simulink model "SF049A_LoaMgr"  (R2013b)
settings: Solver=FixedStepDiscrete  SolverMode=SingleTasking  StartTime=0.0  StopTime=1  FixedStep=0.002  RelTol=1e-3
undefined symbols (not defined in the file): CURRMEASLOAMTGTNMASK_CNT_U08, IVTRLOAMTGTNMASK_CNT_U08, LoaCtrldShtdwn, LoaCurrMeasIdptSigNrFlt, LoaHwTqIdptSigNrFlt, LoaImdtShtdwn, LoaIvtrIdptSigNrFlt, LOAMAXSLEW_ULSPERSEC_F32, LoaMgrCurrIvtrMtgtnRate, LoaMgrCurrIvtrMtgtnSca, LoaMgrCurrIvtrMtgtnScaZeroEna, LoaMgrCurrMeasIdptSig0Resp, LoaMgrCurrMeasIdptSig1Resp, LoaMgrCurrMeasIdptSig2Resp, LoaMgrCurrMeasIdptSigFltThd, LoaMgrCurrMeasMtgtnRate, LoaMgrCurrMeasMtgtnSca, LoaMgrCurrMeasMtgtnScaZeroEna, LoaMgrFadeOutStRate, LoaMgrHwTqIdptSig0NoTqLoaResp, LoaMgrHwTqIdptSig1NoTqLoaResp, LoaMgrHwTqIdptSig2Resp, LoaMgrHwTqIdptSig4Resp, LoaMgrHwTqIdptSigFltThd, LoaMgrHwTqLoaAvlResp, LoaMgrIvtrIdptSig0Resp, LoaMgrIvtrIdptSig1Resp, LoaMgrIvtrIdptSig2Resp, LoaMgrIvtrIdptSigFltThd, LoaMgrIvtrMtgtnRate, LoaMgrIvtrMtgtnSca, LoaMgrIvtrMtgtnScaZeroEna, LoaMgrLimdStRate, LoaMgrLimdStSca, LoaMgrMotAgAvlSnsrlsResp, LoaMgrMotAgIdptSig0NoSnsrlsResp, LoaMgrMotAgIdptSig1NoSnsrlsResp, LoaMgrMotAgIdptSig2Resp, LoaMgrMotAgIdptSig3Resp, LoaMgrMotAgIdptSigFltThd, LoaMgrMotAgMtgtnRate, LoaMgrMotAgMtgtnSca, LoaMgrMotAgMtgtnScaZeroEna, LoaMotAgIdptSigNrFlt, LOASCAONE_ULS_F32, LOASCAZERO_ULS_F32, LoaSt1, LOASTIMDTSHTDWN_CNT_U08, LOASTNORM_CNT_U08, LOASTSWMTGTN_CNT_U08, MAXCURRMEASIDPTSIGALLWD_CNT_U08, MAXHWTQIDPTSIGALLWD_CNT_U08, MAXIVTRIDPTSIGALLWD_CNT_U08, MAXMOTAGMECLIDPTSIGALLWD_CNT_U08, NODEBSTEP_CNT_U16, NtcSts1, SigQlfr1
libraries: simulink x30, NxtrMin x4, NxtrMax x4, NxtrLim x2
(part 4 of 7)

== system SF049A_LoaMgr/LoaMgr/LoaMgrPer1/Arbitrate_Responses/SelFinalResp ==
  note: Pick the most severe of all the requested responses.
      |
      | 5 Immediate Shutdown  (most severe)
      | 4 Controlled Shutdown
      | 3 FadeOut
      | 2 Software-based Mitigation
      | 1 Reduced Performance
      | 0 Normal Operation       (least severe)
  note: Set case 5 as the default.
  MultiMtgtnResp : Inport  RequirementInfo="{'linktype_rmi_doors' '00012fd5 (/E-STEER Core/SubSystem Specifications/Application Functions - EA4/SF049A Loss of Assist Manager)' '#SF049A_145' 'true' 'REQ:  SF049A_145' '' } %GIDa_0bea4813_eb32_4058_8f76_4a113310606c"
  HwTqResp : Inport  RequirementInfo="{'linktype_rmi_doors' '00012fd5 (/E-STEER Core/SubSystem Specifications/Application Functions - EA4/SF049A Loss of Assist Manager)' '#SF049A_145' 'true' 'REQ:  SF049A_145' '' } %GIDa_fb7392d9_74f6_4982_b9b2_ff40e0228010"  Port=2
  MotAgResp : Inport  RequirementInfo="{'linktype_rmi_doors' '00012fd5 (/E-STEER Core/SubSystem Specifications/Application Functions - EA4/SF049A Loss of Assist Manager)' '#SF049A_145' 'true' 'REQ:  SF049A_145' '' } %GIDa_e26ca98c_5988_46fe_9836_793f54528b6a"  Port=3
  CurrMeasResp : Inport  RequirementInfo="{'linktype_rmi_doors' '00012fd5 (/E-STEER Core/SubSystem Specifications/Application Functions - EA4/SF049A Loss of Assist Manager)' '#SF049A_145' 'true' 'REQ:  SF049A_145' '' } %GIDa_907ff0d5_2f07_4379_9f02_e91fd766cda4"  Port=4
  IvtrResp : Inport  RequirementInfo="{'linktype_rmi_doors' '00012fd5 (/E-STEER Core/SubSystem Specifications/Application Functions - EA4/SF049A Loss of Assist Manager)' '#SF049A_145' 'true' 'REQ:  SF049A_145' '' } %GIDa_a6dc34e3_dd60_490f_b49f_75bf24068ace"  Port=5
  CopyRight2 : Subsystem  Description=|  mask(Copyright Information){none=on}
      | Copyright info block.                                               
      |                                                                     
      | Place copyright information at the top of every subsystem in design.
      mask prompts: none "No parameters"
      mask help: Place copyright information at the top of every subsystem in design.
      mask Display:
      | NxtrConf = 'Nexteer Confidential';
      | 
      | sys = bdroot; %handle for the current model ("system")
      | first = get_param(sys,'Created');
      | first = first(end-3:end);  %year is last four digits
      | 
      | last = get_param(sys,'LastModifiedDate');
      | if isempty(last)
      |     last = datestr(now,'yyyy');
      | else
      |     last = last(end-3:end);
      | end
      | 
      | if strcmp(first,last)
      |     fprintf('%s -- Copyright %s Nexteer',NxtrConf,first)
      | else
      |     fprintf('%s -- %s%s- %s Nexteer',NxtrConf,char(169),first,last)
      | end
  F1 : Subsystem  RequirementInfo="{'linktype_rmi_doors' '00012fd5 (/E-STEER Core/SubSystem Specifications/Application Functions - EA4/SF049A Loss of Assist Manager)' '#SF049A_145' 'true' 'REQ:  SF049A_145' '' } %GIDa_26baa418_02ee_4c94_94ec_57afa27eafa7"  TreatAsAtomicUnit=on
      settings: RTWSystemCode=Inline
  F2 : Subsystem  RequirementInfo="{'linktype_rmi_doors' '00012fd5 (/E-STEER Core/SubSystem Specifications/Application Functions - EA4/SF049A Loss of Assist Manager)' '#SF049A_145' 'true' 'REQ:  SF049A_145' '' } %GIDa_a93a0526_eb3f_4f0b_b6f8_7dc588a044fe"  TreatAsAtomicUnit=on
      settings: RTWSystemCode=Inline
  Fade_Out : Subsystem  RequirementInfo="{'linktype_rmi_doors' '00012fd5 (/E-STEER Core/SubSystem Specifications/Application Functions - EA4/SF049A Loss of Assist Manager)' '#SF049A_145' 'true' 'REQ:  SF049A_145' '' } %GIDa_fc0a88a4_dcfe_49c0_8f9c_8d6ed3ce01df"  TreatAsAtomicUnit=on
      settings: RTWSystemCode=Inline
  Merge : Merge  RequirementInfo="{'linktype_rmi_doors' '00012fd5 (/E-STEER Core/SubSystem Specifications/Application Functions - EA4/SF049A Loss of Assist Manager)' '#SF049A_145' 'true' 'REQ:  SF049A_145' '' } %GIDa_9ab56c35_d21c_4b4a_b590_3735befe6dac"  Inputs=6
  MinMax : MinMax  RequirementInfo="{'linktype_rmi_doors' '00012fd5 (/E-STEER Core/SubSystem Specifications/Application Functions - EA4/SF049A Loss of Assist Manager)' '#SF049A_145' 'true' 'REQ:  SF049A_145' '' } %GIDa_5f8ca26d_8ad7_4687_9d19_265b8d1dd2f9"  Function=max  Inputs=5
  Norm : Subsystem  RequirementInfo="{'linktype_rmi_doors' '00012fd5 (/E-STEER Core/SubSystem Specifications/Application Functions - EA4/SF049A Loss of Assist Manager)' '#SF049A_145' 'true' 'REQ:  SF049A_145' '' } %GIDa_8638a703_770e_4f53_9c00_1b7a50679bdd"  TreatAsAtomicUnit=on
      settings: RTWSystemCode=Inline
  Reduced : Subsystem  RequirementInfo="{'linktype_rmi_doors' '00012fd5 (/E-STEER Core/SubSystem Specifications/Application Functions - EA4/SF049A Loss of Assist Manager)' '#SF049A_145' 'true' 'REQ:  SF049A_145' '' } %GIDa_9eb11e77_0847_4d93_baab_0418f3f160a5"  TreatAsAtomicUnit=on
      settings: RTWSystemCode=Inline
  SwBasd_Mtgtn : Subsystem  RequirementInfo="{'linktype_rmi_doors' '00012fd5 (/E-STEER Core/SubSystem Specifications/Application Functions - EA4/SF049A Loss of Assist Manager)' '#SF049A_145' 'true' 'REQ:  SF049A_145' '' } %GIDa_154c4aad_f183_47fd_8b03_2072d0177703"  TreatAsAtomicUnit=on
      settings: RTWSystemCode=Inline
  Switch Case : SwitchCase  RequirementInfo="{'linktype_rmi_doors' '00012fd5 (/E-STEER Core/SubSystem Specifications/Application Functions - EA4/SF049A Loss of Assist Manager)' '#SF049A_145' 'true' 'REQ:  SF049A_145' '' } %GIDa_8f56d13b_bf0d_4688_a08f_d296f9359794"  CaseConditions={0,1,2,3,4}
  LoaSt : Outport  RequirementInfo="{'linktype_rmi_doors' '00012fd5 (/E-STEER Core/SubSystem Specifications/Application Functions - EA4/SF049A Loss of Assist Manager)' '#SF049A_145' 'true' 'REQ:  SF049A_145' '' } %GIDa_af5a8f62_4330_4ff7_9908_06e813b19260"
  wires:
  F1/1(LoaSt) -> Merge/6
  F2/1(LoaSt) -> Merge/5
  Fade_Out/1(LoaSt) -> Merge/4
  SwBasd_Mtgtn/1(LoaSt) -> Merge/3
  Reduced/1(LoaSt) -> Merge/2
  Norm/1(LoaSt) -> Merge/1
  Switch Case/6 -> F1/Action
  Switch Case/5 -> F2/Action
  Switch Case/4 -> Fade_Out/Action
  Switch Case/3 -> SwBasd_Mtgtn/Action
  Switch Case/2 -> Reduced/Action
  Switch Case/1 -> Norm/Action
  MotAgResp/1 -> MinMax/3
  HwTqResp/1 -> MinMax/2
  CurrMeasResp/1 -> MinMax/4
  IvtrResp/1 -> MinMax/5
  Merge/1 -> LoaSt/1
  MinMax/1 -> Switch Case/1
  MultiMtgtnResp/1 -> MinMax/1

== system SF049A_LoaMgr/LoaMgr/LoaMgrPer1/Assign_Scale/CopyRight2 ==

== system SF049A_LoaMgr/LoaMgr/LoaMgrPer1/Assign_Scale/F1 ==
  F1 : ActionPort  ActionType=else
  Constant1 : Constant  Value=LOASCAZERO_ULS_F32
  Constant2 : Constant  Value=LOAMAXSLEW_ULSPERSEC_F32
  CopyRight2 : Subsystem  Description=|  mask(Copyright Information){none=on}
      | Copyright info block.                                               
      |                                                                     
      | Place copyright information at the top of every subsystem in design.
      mask prompts: none "No parameters"
      mask help: Place copyright information at the top of every subsystem in design.
      mask Display:
      | NxtrConf = 'Nexteer Confidential';
      | 
      | sys = bdroot; %handle for the current model ("system")
      | first = get_param(sys,'Created');
      | first = first(end-3:end);  %year is last four digits
      | 
      | last = get_param(sys,'LastModifiedDate');
      | if isempty(last)
      |     last = datestr(now,'yyyy');
      | else
      |     last = last(end-3:end);
      | end
      | 
      | if strcmp(first,last)
      |     fprintf('%s -- Copyright %s Nexteer',NxtrConf,first)
      | else
      |     fprintf('%s -- %s%s- %s Nexteer',NxtrConf,char(169),first,last)
      | end
  Sca : Outport
  Rate : Outport  Port=2
  wires:
  Constant2/1 -> Rate/1
  Constant1/1 -> Sca/1

== system SF049A_LoaMgr/LoaMgr/LoaMgrPer1/Assign_Scale/F2 ==
  F2 : ActionPort  ActionType=elseif
  Constant1 : Constant  Value=LOASCAZERO_ULS_F32
  Constant2 : Constant  Value=LOAMAXSLEW_ULSPERSEC_F32
  CopyRight2 : Subsystem  Description=|  mask(Copyright Information){none=on}
      | Copyright info block.                                               
      |                                                                     
      | Place copyright information at the top of every subsystem in design.
      mask prompts: none "No parameters"
      mask help: Place copyright information at the top of every subsystem in design.
      mask Display:
      | NxtrConf = 'Nexteer Confidential';
      | 
      | sys = bdroot; %handle for the current model ("system")
      | first = get_param(sys,'Created');
      | first = first(end-3:end);  %year is last four digits
      | 
      | last = get_param(sys,'LastModifiedDate');
      | if isempty(last)
      |     last = datestr(now,'yyyy');
      | else
      |     last = last(end-3:end);
      | end
      | 
      | if strcmp(first,last)
      |     fprintf('%s -- Copyright %s Nexteer',NxtrConf,first)
      | else
      |     fprintf('%s -- %s%s- %s Nexteer',NxtrConf,char(169),first,last)
      | end
  Sca : Outport
  Rate : Outport  Port=2
  wires:
  Constant2/1 -> Rate/1
  Constant1/1 -> Sca/1

== system SF049A_LoaMgr/LoaMgr/LoaMgrPer1/Assign_Scale/Fade ==
  Fade : ActionPort  ActionType=elseif
  Constant1 : Constant  Value=LOASCAZERO_ULS_F32
  Constant2 : Constant  Value=LoaMgrFadeOutStRate
  CopyRight2 : Subsystem  Description=|  mask(Copyright Information){none=on}
      | Copyright info block.                                               
      |                                                                     
      | Place copyright information at the top of every subsystem in design.
      mask prompts: none "No parameters"
      mask help: Place copyright information at the top of every subsystem in design.
      mask Display:
      | NxtrConf = 'Nexteer Confidential';
      | 
      | sys = bdroot; %handle for the current model ("system")
      | first = get_param(sys,'Created');
      | first = first(end-3:end);  %year is last four digits
      | 
      | last = get_param(sys,'LastModifiedDate');
      | if isempty(last)
      |     last = datestr(now,'yyyy');
      | else
      |     last = last(end-3:end);
      | end
      | 
      | if strcmp(first,last)
      |     fprintf('%s -- Copyright %s Nexteer',NxtrConf,first)
      | else
      |     fprintf('%s -- %s%s- %s Nexteer',NxtrConf,char(169),first,last)
      | end
  Sca : Outport
  Rate : Outport  Port=2
  wires:
  Constant2/1 -> Rate/1
  Constant1/1 -> Sca/1

== system SF049A_LoaMgr/LoaMgr/LoaMgrPer1/Assign_Scale/Limd ==
  Reduced : ActionPort  ActionType=elseif
  Constant1 : Constant  Value=LoaMgrLimdStSca
  Constant2 : Constant  Value=LoaMgrLimdStRate
  CopyRight2 : Subsystem  Description=|  mask(Copyright Information){none=on}
      | Copyright info block.                                               
      |                                                                     
      | Place copyright information at the top of every subsystem in design.
      mask prompts: none "No parameters"
      mask help: Place copyright information at the top of every subsystem in design.
      mask Display:
      | NxtrConf = 'Nexteer Confidential';
      | 
      | sys = bdroot; %handle for the current model ("system")
      | first = get_param(sys,'Created');
      | first = first(end-3:end);  %year is last four digits
      | 
      | last = get_param(sys,'LastModifiedDate');
      | if isempty(last)
      |     last = datestr(now,'yyyy');
      | else
      |     last = last(end-3:end);
      | end
      | 
      | if strcmp(first,last)
      |     fprintf('%s -- Copyright %s Nexteer',NxtrConf,first)
      | else
      |     fprintf('%s -- %s%s- %s Nexteer',NxtrConf,char(169),first,last)
      | end
  Sca : Outport
  Rate : Outport  Port=2
  wires:
  Constant2/1 -> Rate/1
  Constant1/1 -> Sca/1

== system SF049A_LoaMgr/LoaMgr/LoaMgrPer1/Assign_Scale/Norm ==
  Normal : ActionPort  ActionType=then
  Constant1 : Constant  Value=LOASCAONE_ULS_F32
  Constant2 : Constant  Value=LOAMAXSLEW_ULSPERSEC_F32
  CopyRight2 : Subsystem  Description=|  mask(Copyright Information){none=on}
      | Copyright info block.                                               
      |                                                                     
      | Place copyright information at the top of every subsystem in design.
      mask prompts: none "No parameters"
      mask help: Place copyright information at the top of every subsystem in design.
      mask Display:
      | NxtrConf = 'Nexteer Confidential';
      | 
      | sys = bdroot; %handle for the current model ("system")
      | first = get_param(sys,'Created');
      | first = first(end-3:end);  %year is last four digits
      | 
      | last = get_param(sys,'LastModifiedDate');
      | if isempty(last)
      |     last = datestr(now,'yyyy');
      | else
      |     last = last(end-3:end);
      | end
      | 
      | if strcmp(first,last)
      |     fprintf('%s -- Copyright %s Nexteer',NxtrConf,first)
      | else
      |     fprintf('%s -- %s%s- %s Nexteer',NxtrConf,char(169),first,last)
      | end
  Sca : Outport
  Rate : Outport  Port=2
  wires:
  Constant2/1 -> Rate/1
  Constant1/1 -> Sca/1

== system SF049A_LoaMgr/LoaMgr/LoaMgrPer1/Assign_Scale/SwMtgtn ==
  SwMtgtnEn : Inport
  SwMtgtn : ActionPort  ActionType=elseif
  CopyRight2 : Subsystem  Description=|  mask(Copyright Information){none=on}
      | Copyright info block.                                               
      |                                                                     
      | Place copyright information at the top of every subsystem in design.
      mask prompts: none "No parameters"
      mask help: Place copyright information at the top of every subsystem in design.
      mask Display:
      | NxtrConf = 'Nexteer Confidential';
      | 
      | sys = bdroot; %handle for the current model ("system")
      | first = get_param(sys,'Created');
      | first = first(end-3:end);  %year is last four digits
      | 
      | last = get_param(sys,'LastModifiedDate');
      | if isempty(last)
      |     last = datestr(now,'yyyy');
      | else
      |     last = last(end-3:end);
      | end
      | 
      | if strcmp(first,last)
      |     fprintf('%s -- Copyright %s Nexteer',NxtrConf,first)
      | else
      |     fprintf('%s -- %s%s- %s Nexteer',NxtrConf,char(169),first,last)
      | end
  Data Store Read1 : DataStoreRead  Priority=1  DataStoreName=PrevVltgModSrc
  Data Store Read3 : DataStoreRead  RequirementInfo="{'linktype_rmi_doors' '00012fd5 (/E-STEER Core/SubSystem Specifications/Application Functions - EA4/SF049A Loss of Assist Manager)' '#SF049A_155' 'true' 'REQ:  SF049A_155' '' } %GIDa_3c546dda_ea9f_49a0_aeea_eabfc17e49f2"  Priority=1  DataStoreName=PrevMotAgLoaMtgtnEna
  Data Store Write1 : DataStoreWrite  Priority=2  DataStoreName=PrevVltgModSrc
  Data Store Write2 : DataStoreWrite  Priority=2  DataStoreName=PrevMotAgLoaMtgtnEna
  Demux : Demux
  HwTqTrue : Subsystem  RequirementInfo="{'linktype_rmi_doors' '00012fd5 (/E-STEER Core/SubSystem Specifications/Application Functions - EA4/SF049A Loss of Assist Manager)' '#SF049A_154' 'true' 'REQ:  SF049A_154' '' } %GIDa_62d381ba_13cd_4ede_a80b_d2d2bbee5c07"  TreatAsAtomicUnit=on
      settings: RTWSystemCode=Inline
  If : If  RequirementInfo="{'linktype_rmi_doors' '00012fd5 (/E-STEER Core/SubSystem Specifications/Application Functions - EA4/SF049A Loss of Assist Manager)' '#SF049A_154' 'true' 'REQ:  SF049A_154' '' ; 'linktype_rmi_doors' '00012fd5 (/E-STEER Core/SubSystem Specifications/Application Functions - EA4/SF049A Loss of Assist Manager)' '#SF049A_155' 'true' 'REQ:  SF049A_155' '' ; 'linktype_rmi_doors' '00012fd5 (/E-STEER Core/SubSystem Specifications/Application Functions - EA4/SF049A Loss of Assist Manager)' '#SF049A_156' 'true' 'REQ:  SF049A_156' '' } %GIDa_75fd0f55_6e5a_43cb_bf82_5549743f4a47"  NumInputs=2  IfExpression=u1  ElseIfExpressions=u2
  MaskBooleans : Subsystem  RequirementInfo="{'linktype_rmi_doors' '00012fd5 (/E-STEER Core/SubSystem Specifications/Application Functions - EA4/SF049A Loss of Assist Manager)' '#SF049A_156' 'true' 'REQ:  SF049A_156' '' } %GIDa_9ee9f9da_0779_4fcb_b968_b795a26852c5"
  Merge : Merge  RequirementInfo="{'linktype_rmi_doors' '00012fd5 (/E-STEER Core/SubSystem Specifications/Application Functions - EA4/SF049A Loss of Assist Manager)' '#SF049A_154' 'true' 'REQ:  SF049A_154' '' ; 'linktype_rmi_doors' '00012fd5 (/E-STEER Core/SubSystem Specifications/Application Functions - EA4/SF049A Loss of Assist Manager)' '#SF049A_155' 'true' 'REQ:  SF049A_155' '' ; 'linktype_rmi_doors' '00012fd5 (/E-STEER Core/SubSystem Specifications/Application Functions - EA4/SF049A Loss of Assist Manager)' '#SF049A_156' 'true' 'REQ:  SF049A_156' '' } %GIDa_eed0bbff_a26b_467a_b875_5188c4c7366d"  Inputs=3
  Merge1 : Merge  RequirementInfo="{'linktype_rmi_doors' '00012fd5 (/E-STEER Core/SubSystem Specifications/Application Functions - EA4/SF049A Loss of Assist Manager)' '#SF049A_154' 'true' 'REQ:  SF049A_154' '' ; 'linktype_rmi_doors' '00012fd5 (/E-STEER Core/SubSystem Specifications/Application Functions - EA4/SF049A Loss of Assist Manager)' '#SF049A_155' 'true' 'REQ:  SF049A_155' '' ; 'linktype_rmi_doors' '00012fd5 (/E-STEER Core/SubSystem Specifications/Application Functions - EA4/SF049A Loss of Assist Manager)' '#SF049A_156' 'true' 'REQ:  SF049A_156' '' } %GIDa_825d185b_3837_4a2c_882e_4a3b520e55db"  Inputs=3
  MotAgTrue : Subsystem  RequirementInfo="{'linktype_rmi_doors' '00012fd5 (/E-STEER Core/SubSystem Specifications/Application Functions - EA4/SF049A Loss of Assist Manager)' '#SF049A_155' 'true' 'REQ:  SF049A_155' '' } %GIDa_b6733dae_63ac_4bee_b8f5_33763c360099"  TreatAsAtomicUnit=on
      settings: RTWSystemCode=Inline
  OthersTrue : Subsystem  RequirementInfo="{'linktype_rmi_doors' '00012fd5 (/E-STEER Core/SubSystem Specifications/Application Functions - EA4/SF049A Loss of Assist Manager)' '#SF049A_156' 'true' 'REQ:  SF049A_156' '' } %GIDa_3cccd697_8f6b_4aaa_9530_e4cc0996cd34"  TreatAsAtomicUnit=on
      settings: RTWSystemCode=Inline
  Sca : Outport  RequirementInfo={} %GIDa_7428dcfa_fbc4_4f9a_a71c_552d563de483
  Rate : Outport  RequirementInfo={} %GIDa_89a5bc68_6e8b_4db9_b4fd_e79c8200b00d  Port=2
  wires:
  Merge1/1 -> Rate/1
  Merge/1 -> Sca/1
  OthersTrue/2(Rate) -> Merge1/3
  OthersTrue/1(Sca) -> Merge/3
  MotAgTrue/2(Rate) -> Merge1/2
  HwTqTrue/2(Rate) -> Merge1/1
  MotAgTrue/1(Sca) -> Merge/2
  HwTqTrue/1(Sca) -> Merge/1
  Data Store Read1/1 -> OthersTrue/2(PrevVltgModSrc)
  MaskBooleans/1(VltgModSrc) -> Data Store Write1/1, OthersTrue/1(VltgModSrc)
  If/3 -> OthersTrue/Action
  Data Store Read3/1 -> MotAgTrue/1(PrevMotAgLoaMtgtnEn)
  If/2 -> MotAgTrue/Action
  If/1 -> HwTqTrue/Action
  Demux/4 -> MaskBooleans/2(IvtrLoaMtgtnEna)  "IvtrLoaMtgtnEna"
  Demux/3 -> MaskBooleans/1(CurrMeasLoaMtgtnEna)  "CurrMeasLoaMtgtnEna"
  Demux/2 -> If/2, Data Store Write2/1  "MotAgLoaMtgtnEna"
  Demux/1 -> If/1  "HwTqLoaMtgtnEna"
  SwMtgtnEn/1 -> Demux/1

== system SF049A_LoaMgr/LoaMgr/LoaMgrPer1/Calc_Ivtr_State/CopyRight2 ==

== system SF049A_LoaMgr/LoaMgr/LoaMgrPer1/Calc_Ivtr_State/Ivtr1Sts_ELSE ==
  In1 : Inport
  Action Port : ActionPort  ActionType=else
  CopyRight2 : Subsystem  Description=|  mask(Copyright Information){none=on}
      | Copyright info block.                                               
      |                                                                     
      | Place copyright information at the top of every subsystem in design.
      mask prompts: none "No parameters"
      mask help: Place copyright information at the top of every subsystem in design.
      mask Display:
      | NxtrConf = 'Nexteer Confidential';
      | 
      | sys = bdroot; %handle for the current model ("system")
      | first = get_param(sys,'Created');
      | first = first(end-3:end);  %year is last four digits
      | 
      | last = get_param(sys,'LastModifiedDate');
      | if isempty(last)
      |     last = datestr(now,'yyyy');
      | else
      |     last = last(end-3:end);
      | end
      | 
      | if strcmp(first,last)
      |     fprintf('%s -- Copyright %s Nexteer',NxtrConf,first)
      | else
      |     fprintf('%s -- %s%s- %s Nexteer',NxtrConf,char(169),first,last)
      | end
  Out1 : Outport
  wires:
  In1/1 -> Out1/1

== system SF049A_LoaMgr/LoaMgr/LoaMgrPer1/Calc_Ivtr_State/Ivtr1Sts_THEN ==
  In1 : Inport
  Action Port : ActionPort  ActionType=then
  CopyRight2 : Subsystem  Description=|  mask(Copyright Information){none=on}
      | Copyright info block.                                               
      |                                                                     
      | Place copyright information at the top of every subsystem in design.
      mask prompts: none "No parameters"
      mask help: Place copyright information at the top of every subsystem in design.
      mask Display:
      | NxtrConf = 'Nexteer Confidential';
      | 
      | sys = bdroot; %handle for the current model ("system")
      | first = get_param(sys,'Created');
      | first = first(end-3:end);  %year is last four digits
      | 
      | last = get_param(sys,'LastModifiedDate');
      | if isempty(last)
      |     last = datestr(now,'yyyy');
      | else
      |     last = last(end-3:end);
      | end
      | 
      | if strcmp(first,last)
      |     fprintf('%s -- Copyright %s Nexteer',NxtrConf,first)
      | else
      |     fprintf('%s -- %s%s- %s Nexteer',NxtrConf,char(169),first,last)
      | end
  Out2 : Outport
  wires:
  In1/1 -> Out2/1

== system SF049A_LoaMgr/LoaMgr/LoaMgrPer1/Calc_Ivtr_State/Ivtr2Sts_ELSE ==
  In1 : Inport
  Action Port : ActionPort  ActionType=else
  CopyRight2 : Subsystem  Description=|  mask(Copyright Information){none=on}
      | Copyright info block.                                               
      |                                                                     
      | Place copyright information at the top of every subsystem in design.
      mask prompts: none "No parameters"
      mask help: Place copyright information at the top of every subsystem in design.
      mask Display:
      | NxtrConf = 'Nexteer Confidential';
      | 
      | sys = bdroot; %handle for the current model ("system")
      | first = get_param(sys,'Created');
      | first = first(end-3:end);  %year is last four digits
      | 
      | last = get_param(sys,'LastModifiedDate');
      | if isempty(last)
      |     last = datestr(now,'yyyy');
      | else
      |     last = last(end-3:end);
      | end
      | 
      | if strcmp(first,last)
      |     fprintf('%s -- Copyright %s Nexteer',NxtrConf,first)
      | else
      |     fprintf('%s -- %s%s- %s Nexteer',NxtrConf,char(169),first,last)
      | end
  Out1 : Outport
  wires:
  In1/1 -> Out1/1

== system SF049A_LoaMgr/LoaMgr/LoaMgrPer1/Calc_Ivtr_State/Ivtr2Sts_THEN ==
  In1 : Inport
  Action Port : ActionPort  ActionType=then
  CopyRight2 : Subsystem  Description=|  mask(Copyright Information){none=on}
      | Copyright info block.                                               
      |                                                                     
      | Place copyright information at the top of every subsystem in design.
      mask prompts: none "No parameters"
      mask help: Place copyright information at the top of every subsystem in design.
      mask Display:
      | NxtrConf = 'Nexteer Confidential';
      | 
      | sys = bdroot; %handle for the current model ("system")
      | first = get_param(sys,'Created');
      | first = first(end-3:end);  %year is last four digits
      | 
      | last = get_param(sys,'LastModifiedDate');
      | if isempty(last)
      |     last = datestr(now,'yyyy');
      | else
      |     last = last(end-3:end);
      | end
      | 
      | if strcmp(first,last)
      |     fprintf('%s -- Copyright %s Nexteer',NxtrConf,first)
      | else
      |     fprintf('%s -- %s%s- %s Nexteer',NxtrConf,char(169),first,last)
      | end
  Out1 : Outport
  wires:
  In1/1 -> Out1/1

== system SF049A_LoaMgr/LoaMgr/LoaMgrPer1/Latch_Inputs/CopyRight2 ==

== system SF049A_LoaMgr/LoaMgr/LoaMgrPer1/Latch_Inputs/RngLimCurrMeasIdptSig ==
  CurrMeasIdptSig : Inport  RequirementInfo="{'linktype_rmi_doors' '00012fd5 (/E-STEER Core/SubSystem Specifications/Application Functions - EA4/SF049A Loss of Assist Manager)' '#SF049A_116' 'true' 'REQ:  SF049A_116' '' } %GIDa_9625436b_77ac_4feb_94b8_691fb9249b94"
  " 1" : Merge  RequirementInfo="{'linktype_rmi_doors' '00012fd5 (/E-STEER Core/SubSystem Specifications/Application Functions - EA4/SF049A Loss of Assist Manager)' '#SF049A_116' 'true' 'REQ:  SF049A_116' '' } %GIDa_158bc258_ef4d_455e_8502_48ed43592478"
  Allw : Subsystem  RequirementInfo="{'linktype_rmi_doors' '00012fd5 (/E-STEER Core/SubSystem Specifications/Application Functions - EA4/SF049A Loss of Assist Manager)' '#SF049A_116' 'true' 'REQ:  SF049A_116' '' } %GIDa_dd4cc193_4217_49cf_b9a4_07f044e8a2c9"  TreatAsAtomicUnit=on
      settings: RTWSystemCode=Inline
  Compare To Constant1 : simulink/Logic and Bit Operations/Compare To Constant  RequirementInfo="{'linktype_rmi_doors' '00012fd5 (/E-STEER Core/SubSystem Specifications/Application Functions - EA4/SF049A Loss of Assist Manager)' '#SF049A_116' 'true' 'REQ:  SF049A_116' '' } %GIDa_b6bd0f19_3e46_460e_b9d9_b3470dce084f"  relop=>  const=MAXCURRMEASIDPTSIGALLWD_CNT_U08  OutDataTypeStr=boolean
  Constant2 : Constant  RequirementInfo="{'linktype_rmi_doors' '00012fd5 (/E-STEER Core/SubSystem Specifications/Application Functions - EA4/SF049A Loss of Assist Manager)' '#SF049A_116' 'true' 'REQ:  SF049A_116' '' } %GIDa_ca24a87a_b587_459e_b57e_7ef8f1b2aa36"  Value=0  OutDataTypeStr=uint8
      settings: AttributesFormatString=%<OutDataTypeStr>
  CopyRight2 : Subsystem  Description=|  mask(Copyright Information){none=on}
      | Copyright info block.                                               
      |                                                                     
      | Place copyright information at the top of every subsystem in design.
      mask prompts: none "No parameters"
      mask help: Place copyright information at the top of every subsystem in design.
      mask Display:
      | NxtrConf = 'Nexteer Confidential';
      | 
      | sys = bdroot; %handle for the current model ("system")
      | first = get_param(sys,'Created');
      | first = first(end-3:end);  %year is last four digits
      | 
      | last = get_param(sys,'LastModifiedDate');
      | if isempty(last)
      |     last = datestr(now,'yyyy');
      | else
      |     last = last(end-3:end);
      | end
      | 
      | if strcmp(first,last)
      |     fprintf('%s -- Copyright %s Nexteer',NxtrConf,first)
      | else
      |     fprintf('%s -- %s%s- %s Nexteer',NxtrConf,char(169),first,last)
      | end
  DftVal : Subsystem  RequirementInfo="{'linktype_rmi_doors' '00012fd5 (/E-STEER Core/SubSystem Specifications/Application Functions - EA4/SF049A Loss of Assist Manager)' '#SF049A_116' 'true' 'REQ:  SF049A_116' '' } %GIDa_2d8e1074_7936_4c50_aee5_f2889c060ad6"  TreatAsAtomicUnit=on
      settings: RTWSystemCode=Inline
  Ivtr1Inactv_IF1 : If  RequirementInfo="{'linktype_rmi_doors' '00012fd5 (/E-STEER Core/SubSystem Specifications/Application Functions - EA4/SF049A Loss of Assist Manager)' '#SF049A_116' 'true' 'REQ:  SF049A_116' '' } %GIDa_e866b207_0d86_4aa2_b3a5_8045b8063649"  IfExpression=u1
  RngLimdCurrMeasIdptSig : Outport  RequirementInfo="{'linktype_rmi_doors' '00012fd5 (/E-STEER Core/SubSystem Specifications/Application Functions - EA4/SF049A Loss of Assist Manager)' '#SF049A_116' 'true' 'REQ:  SF049A_116' '' } %GIDa_45d348bd_2c86_4526_9088_eae6dc9fb1ad"
  wires:
  Compare To Constant1/1 -> Ivtr1Inactv_IF1/1
  Allw/1(Out1) -> " 1"/2
  Constant2/1 -> DftVal/1(In1)
  " 1"/1 -> RngLimdCurrMeasIdptSig/1
  DftVal/1(Out2) -> " 1"/1
  Ivtr1Inactv_IF1/2 -> Allw/Action
  Ivtr1Inactv_IF1/1 -> DftVal/Action
  CurrMeasIdptSig/1 -> Compare To Constant1/1, Allw/1(In1)

== system SF049A_LoaMgr/LoaMgr/LoaMgrPer1/Latch_Inputs/RngLimHwTqIdptSig ==
  HwTqIdptSig : Inport  RequirementInfo="{'linktype_rmi_doors' '00012fd5 (/E-STEER Core/SubSystem Specifications/Application Functions - EA4/SF049A Loss of Assist Manager)' '#SF049A_112' 'true' 'REQ:  SF049A_112' '' } %GIDa_7863f3d6_b5d2_4bbd_84c3_64f9f5a9e6a9"
  " 1" : Merge  RequirementInfo="{'linktype_rmi_doors' '00012fd5 (/E-STEER Core/SubSystem Specifications/Application Functions - EA4/SF049A Loss of Assist Manager)' '#SF049A_112' 'true' 'REQ:  SF049A_112' '' } %GIDa_6b30d1d0_3193_45c0_9adc_491dc9bc89b4"
  Allw : Subsystem  RequirementInfo="{'linktype_rmi_doors' '00012fd5 (/E-STEER Core/SubSystem Specifications/Application Functions - EA4/SF049A Loss of Assist Manager)' '#SF049A_112' 'true' 'REQ:  SF049A_112' '' } %GIDa_c633fbd2_8136_4d6a_92c3_c490fa414dee"  TreatAsAtomicUnit=on
      settings: RTWSystemCode=Inline
  Compare To Constant1 : simulink/Logic and Bit Operations/Compare To Constant  RequirementInfo="{'linktype_rmi_doors' '00012fd5 (/E-STEER Core/SubSystem Specifications/Application Functions - EA4/SF049A Loss of Assist Manager)' '#SF049A_112' 'true' 'REQ:  SF049A_112' '' } %GIDa_30ceeeba_5c72_4564_b644_fe09951d0984"  relop=>  const=MAXHWTQIDPTSIGALLWD_CNT_U08  OutDataTypeStr=boolean
  Constant2 : Constant  RequirementInfo="{'linktype_rmi_doors' '00012fd5 (/E-STEER Core/SubSystem Specifications/Application Functions - EA4/SF049A Loss of Assist Manager)' '#SF049A_112' 'true' 'REQ:  SF049A_112' '' } %GIDa_2e9d68eb_4030_4298_989a_79fb00f4b2a4"  Value=0  OutDataTypeStr=uint8
      settings: AttributesFormatString=%<OutDataTypeStr>
  CopyRight2 : Subsystem  Description=|  mask(Copyright Information){none=on}
      | Copyright info block.                                               
      |                                                                     
      | Place copyright information at the top of every subsystem in design.
      mask prompts: none "No parameters"
      mask help: Place copyright information at the top of every subsystem in design.
      mask Display:
      | NxtrConf = 'Nexteer Confidential';
      | 
      | sys = bdroot; %handle for the current model ("system")
      | first = get_param(sys,'Created');
      | first = first(end-3:end);  %year is last four digits
      | 
      | last = get_param(sys,'LastModifiedDate');
      | if isempty(last)
      |     last = datestr(now,'yyyy');
      | else
      |     last = last(end-3:end);
      | end
      | 
      | if strcmp(first,last)
      |     fprintf('%s -- Copyright %s Nexteer',NxtrConf,first)
      | else
      |     fprintf('%s -- %s%s- %s Nexteer',NxtrConf,char(169),first,last)
      | end
  DftVal : Subsystem  RequirementInfo="{'linktype_rmi_doors' '00012fd5 (/E-STEER Core/SubSystem Specifications/Application Functions - EA4/SF049A Loss of Assist Manager)' '#SF049A_112' 'true' 'REQ:  SF049A_112' '' } %GIDa_192a1aa3_c915_4d4c_8f5f_684b45fc2133"  TreatAsAtomicUnit=on
      settings: RTWSystemCode=Inline
  Ivtr1Inactv_IF1 : If  RequirementInfo="{'linktype_rmi_doors' '00012fd5 (/E-STEER Core/SubSystem Specifications/Application Functions - EA4/SF049A Loss of Assist Manager)' '#SF049A_112' 'true' 'REQ:  SF049A_112' '' } %GIDa_e7da3207_7a73_4cf5_8725_957c0865fca6"  IfExpression=u1
  RngLimdHwTqIdptSig : Outport  RequirementInfo="{'linktype_rmi_doors' '00012fd5 (/E-STEER Core/SubSystem Specifications/Application Functions - EA4/SF049A Loss of Assist Manager)' '#SF049A_112' 'true' 'REQ:  SF049A_112' '' } %GIDa_aa1c36d8_2247_4ae6_86fe_70666c1dd457"
  wires:
  Compare To Constant1/1 -> Ivtr1Inactv_IF1/1
  Allw/1(Out1) -> " 1"/2
  Constant2/1 -> DftVal/1(In1)
  " 1"/1 -> RngLimdHwTqIdptSig/1
  DftVal/1(Out2) -> " 1"/1
  Ivtr1Inactv_IF1/2 -> Allw/Action
  Ivtr1Inactv_IF1/1 -> DftVal/Action
  HwTqIdptSig/1 -> Compare To Constant1/1, Allw/1(In1)

== system SF049A_LoaMgr/LoaMgr/LoaMgrPer1/Latch_Inputs/RngLimMotAgMecIdptSig ==
  MotAgMeclIdptSig : Inport  RequirementInfo="{'linktype_rmi_doors' '00012fd5 (/E-STEER Core/SubSystem Specifications/Application Functions - EA4/SF049A Loss of Assist Manager)' '#SF049A_114' 'true' 'REQ:  SF049A_114' '' } %GIDa_c4f72a4a_986d_4c55_a8ef_b4f4c01c64e7"
  " 1" : Merge  RequirementInfo="{'linktype_rmi_doors' '00012fd5 (/E-STEER Core/SubSystem Specifications/Application Functions - EA4/SF049A Loss of Assist Manager)' '#SF049A_114' 'true' 'REQ:  SF049A_114' '' } %GIDa_72f53818_2c39_4bdd_9729_efb1e66565e9"
  Allw : Subsystem  RequirementInfo="{'linktype_rmi_doors' '00012fd5 (/E-STEER Core/SubSystem Specifications/Application Functions - EA4/SF049A Loss of Assist Manager)' '#SF049A_114' 'true' 'REQ:  SF049A_114' '' } %GIDa_024cc470_5a14_4f9b_85ba_013f2d37bdda"  TreatAsAtomicUnit=on
      settings: RTWSystemCode=Inline
  Compare To Constant1 : simulink/Logic and Bit Operations/Compare To Constant  RequirementInfo="{'linktype_rmi_doors' '00012fd5 (/E-STEER Core/SubSystem Specifications/Application Functions - EA4/SF049A Loss of Assist Manager)' '#SF049A_114' 'true' 'REQ:  SF049A_114' '' } %GIDa_17c2f090_135b_4a7b_ab0f_5292a3d981bb"  relop=>  const=MAXMOTAGMECLIDPTSIGALLWD_CNT_U08  OutDataTypeStr=boolean
  Constant2 : Constant  RequirementInfo="{'linktype_rmi_doors' '00012fd5 (/E-STEER Core/SubSystem Specifications/Application Functions - EA4/SF049A Loss of Assist Manager)' '#SF049A_114' 'true' 'REQ:  SF049A_114' '' } %GIDa_1c9e9e31_3abd_4604_aa0e_41aba5c38795"  Value=0  OutDataTypeStr=uint8
      settings: AttributesFormatString=%<OutDataTypeStr>
  CopyRight2 : Subsystem  Description=|  mask(Copyright Information){none=on}
      | Copyright info block.                                               
      |                                                                     
      | Place copyright information at the top of every subsystem in design.
      mask prompts: none "No parameters"
      mask help: Place copyright information at the top of every subsystem in design.
      mask Display:
      | NxtrConf = 'Nexteer Confidential';
      | 
      | sys = bdroot; %handle for the current model ("system")
      | first = get_param(sys,'Created');
      | first = first(end-3:end);  %year is last four digits
      | 
      | last = get_param(sys,'LastModifiedDate');
      | if isempty(last)
      |     last = datestr(now,'yyyy');
      | else
      |     last = last(end-3:end);
      | end
      | 
      | if strcmp(first,last)
      |     fprintf('%s -- Copyright %s Nexteer',NxtrConf,first)
      | else
      |     fprintf('%s -- %s%s- %s Nexteer',NxtrConf,char(169),first,last)
      | end
  DftVal : Subsystem  RequirementInfo="{'linktype_rmi_doors' '00012fd5 (/E-STEER Core/SubSystem Specifications/Application Functions - EA4/SF049A Loss of Assist Manager)' '#SF049A_114' 'true' 'REQ:  SF049A_114' '' } %GIDa_1748abad_775f_4b87_b4ad_c58cff3316ca"  TreatAsAtomicUnit=on
      settings: RTWSystemCode=Inline
  Ivtr1Inactv_IF1 : If  RequirementInfo="{'linktype_rmi_doors' '00012fd5 (/E-STEER Core/SubSystem Specifications/Application Functions - EA4/SF049A Loss of Assist Manager)' '#SF049A_114' 'true' 'REQ:  SF049A_114' '' } %GIDa_f9be2c60_a56e_451b_8e2c_7381cbdea29f"  IfExpression=u1
  RngLimdMotAgMecIdptSig : Outport  RequirementInfo="{'linktype_rmi_doors' '00012fd5 (/E-STEER Core/SubSystem Specifications/Application Functions - EA4/SF049A Loss of Assist Manager)' '#SF049A_114' 'true' 'REQ:  SF049A_114' '' } %GIDa_001cb7f1_fe75_453f_a829_925ced19f1d5"
  wires:
  MotAgMeclIdptSig/1 -> Allw/1(In1), Compare To Constant1/1
  Ivtr1Inactv_IF1/1 -> DftVal/Action
  Ivtr1Inactv_IF1/2 -> Allw/Action
  DftVal/1(Out2) -> " 1"/1
  " 1"/1 -> RngLimdMotAgMecIdptSig/1
  Constant2/1 -> DftVal/1(In1)
  Allw/1(Out1) -> " 1"/2
  Compare To Constant1/1 -> Ivtr1Inactv_IF1/1

== system SF049A_LoaMgr/LoaMgr/LoaMgrPer1/Request_Responses/CopyRight1 ==

== system SF049A_LoaMgr/LoaMgr/LoaMgrPer1/Request_Responses/CurrMeasResp ==
  note: SWITCH CurrMeasIdptMin
      |     CASE 2
      |         CurrMeasResp = LoaMgrCurrMeasIdptSig2Resp
      |     CASE 1
      |          CurrMeasResp = LoaMgrCurrMeasIdptSig1Resp
      |     CASE ELSE
      |          CurrMeasResp = LoaMgrCurrMeasIdptSig0Resp
      | ENDSWITCH
  CurrMeasIdptMin : Inport  RequirementInfo={} %GIDa_3ebcd9c5_6f25_4d09_87f8_6cb15c7b13b2
  Constant : Constant  RequirementInfo="{'linktype_rmi_doors' '00012fd5 (/E-STEER Core/SubSystem Specifications/Application Functions - EA4/SF049A Loss of Assist Manager)' '#SF049A_126' 'true' 'REQ:  SF049A_126' '' } %GIDa_e62e08bd_cdb2_40a6_bb2f_f57d543256fd"  Value=LoaMgrCurrMeasIdptSig2Resp
  Constant1 : Constant  RequirementInfo="{'linktype_rmi_doors' '00012fd5 (/E-STEER Core/SubSystem Specifications/Application Functions - EA4/SF049A Loss of Assist Manager)' '#SF049A_126' 'true' 'REQ:  SF049A_126' '' } %GIDa_65e39575_48ab_42b9_b787_01ade7a7e64a"  Value=LoaMgrCurrMeasIdptSig1Resp
  Constant2 : Constant  RequirementInfo="{'linktype_rmi_doors' '00012fd5 (/E-STEER Core/SubSystem Specifications/Application Functions - EA4/SF049A Loss of Assist Manager)' '#SF049A_126' 'true' 'REQ:  SF049A_126' '' } %GIDa_fb6bd49e_4660_4ee0_9caa_aeb37d417315"  Value=LoaMgrCurrMeasIdptSig0Resp
  CopyRight2 : Subsystem  Description=|  mask(Copyright Information){none=on}
      | Copyright info block.                                               
      |                                                                     
      | Place copyright information at the top of every subsystem in design.
      mask prompts: none "No parameters"
      mask help: Place copyright information at the top of every subsystem in design.
      mask Display:
      | NxtrConf = 'Nexteer Confidential';
      | 
      | sys = bdroot; %handle for the current model ("system")
      | first = get_param(sys,'Created');
      | first = first(end-3:end);  %year is last four digits
      | 
      | last = get_param(sys,'LastModifiedDate');
      | if isempty(last)
      |     last = datestr(now,'yyyy');
      | else
      |     last = last(end-3:end);
      | end
      | 
      | if strcmp(first,last)
      |     fprintf('%s -- Copyright %s Nexteer',NxtrConf,first)
      | else
      |     fprintf('%s -- %s%s- %s Nexteer',NxtrConf,char(169),first,last)
      | end
  Merge1 : Merge  RequirementInfo="{'linktype_rmi_doors' '00012fd5 (/E-STEER Core/SubSystem Specifications/Application Functions - EA4/SF049A Loss of Assist Manager)' '#SF049A_126' 'true' 'REQ:  SF049A_126' '' } %GIDa_5d4ef986_29fc_405c_a0d0_c4f1ce89bc8b"  Inputs=3
  Switch Case : SwitchCase  RequirementInfo="{'linktype_rmi_doors' '00012fd5 (/E-STEER Core/SubSystem Specifications/Application Functions - EA4/SF049A Loss of Assist Manager)' '#SF049A_126' 'true' 'REQ:  SF049A_126' '' } %GIDa_02add338_e7f3_4153_b7ff_3ce10adcbada"  CaseConditions={2,1}
  Two : Subsystem  RequirementInfo="{'linktype_rmi_doors' '00012fd5 (/E-STEER Core/SubSystem Specifications/Application Functions - EA4/SF049A Loss of Assist Manager)' '#SF049A_126' 'true' 'REQ:  SF049A_126' '' } %GIDa_b296c330_bd21_43f2_a4d3_297be62c676a"  TreatAsAtomicUnit=on
      settings: RTWSystemCode=Inline
  Zero_or_Invalid : Subsystem  RequirementInfo="{'linktype_rmi_doors' '00012fd5 (/E-STEER Core/SubSystem Specifications/Application Functions - EA4/SF049A Loss of Assist Manager)' '#SF049A_126' 'true' 'REQ:  SF049A_126' '' } %GIDa_3a826e90_1dc4_4880_b3cd_ebf9d76bc9f2"  TreatAsAtomicUnit=on
      settings: RTWSystemCode=Inline
  one : Subsystem  RequirementInfo="{'linktype_rmi_doors' '00012fd5 (/E-STEER Core/SubSystem Specifications/Application Functions - EA4/SF049A Loss of Assist Manager)' '#SF049A_126' 'true' 'REQ:  SF049A_126' '' } %GIDa_7ea89eeb_1573_4dbd_8a83_88b85a71b59d"  TreatAsAtomicUnit=on
      settings: RTWSystemCode=Inline
  CurrMeasResp : Outport  RequirementInfo={} %GIDa_56c90ba4_d79b_4181_842e_b679ad2a0347
  wires:
  Constant2/1 -> Zero_or_Invalid/1(Sig0Resp)
  Zero_or_Invalid/1(CurrMeasResp) -> Merge1/3
  Merge1/1 -> CurrMeasResp/1
  one/1(CurrMeasResp) -> Merge1/2
  Two/1(CurrMeasResp) -> Merge1/1
  Constant1/1 -> one/1(Sig1Resp)
  Switch Case/2 -> one/Action
  Constant/1 -> Two/1(Sig2Resp)
  Switch Case/1 -> Two/Action
  Switch Case/3 -> Zero_or_Invalid/Action
  CurrMeasIdptMin/1 -> Switch Case/1

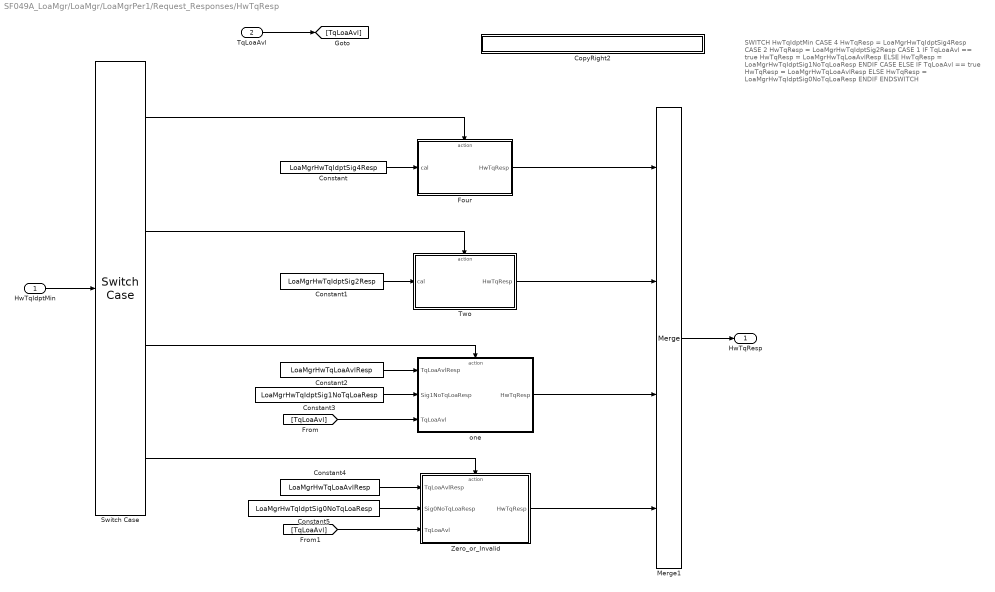
== system SF049A_LoaMgr/LoaMgr/LoaMgrPer1/Request_Responses/HwTqResp ==
  note: SWITCH HwTqIdptMin
      |     CASE 4
      |         HwTqResp = LoaMgrHwTqIdptSig4Resp
      |     CASE 2
      |         HwTqResp = LoaMgrHwTqIdptSig2Resp
      |     CASE 1
      |         IF TqLoaAvl == true
      |             HwTqResp = LoaMgrHwTqLoaAvlResp
      |         ELSE
      |             HwTqResp = LoaMgrHwTqIdptSig1NoTqLoaResp
      |         ENDIF
      |     CASE ELSE
      |         IF TqLoaAvl == true
      |             HwTqResp = LoaMgrHwTqLoaAvlResp
      |         ELSE
      |             HwTqResp = LoaMgrHwTqIdptSig0NoTqLoaResp
      |         ENDIF
      | ENDSWITCH
  HwTqIdptMin : Inport
  TqLoaAvl : Inport  Port=2
  Constant : Constant  RequirementInfo="{'linktype_rmi_doors' '00012fd5 (/E-STEER Core/SubSystem Specifications/Application Functions - EA4/SF049A Loss of Assist Manager)' '#SF049A_120' 'true' 'REQ:  SF049A_120' '' } %GIDa_7c6f5a88_9ab8_4047_b404_ad39e8cff8cc"  Value=LoaMgrHwTqIdptSig4Resp
  Constant1 : Constant  RequirementInfo="{'linktype_rmi_doors' '00012fd5 (/E-STEER Core/SubSystem Specifications/Application Functions - EA4/SF049A Loss of Assist Manager)' '#SF049A_120' 'true' 'REQ:  SF049A_120' '' } %GIDa_99da27c7_ba8b_44ad_855f_6847e09baced"  Value=LoaMgrHwTqIdptSig2Resp
  Constant2 : Constant  RequirementInfo="{'linktype_rmi_doors' '00012fd5 (/E-STEER Core/SubSystem Specifications/Application Functions - EA4/SF049A Loss of Assist Manager)' '#SF049A_120' 'true' 'REQ:  SF049A_120' '' } %GIDa_66b0477f_ff5f_4d1c_a4fe_f74c98e05254"  Value=LoaMgrHwTqLoaAvlResp
  Constant3 : Constant  RequirementInfo="{'linktype_rmi_doors' '00012fd5 (/E-STEER Core/SubSystem Specifications/Application Functions - EA4/SF049A Loss of Assist Manager)' '#SF049A_120' 'true' 'REQ:  SF049A_120' '' } %GIDa_3946beda_73e8_43f1_994b_9c8133215dcc"  Value=LoaMgrHwTqIdptSig1NoTqLoaResp
  Constant4 : Constant  RequirementInfo="{'linktype_rmi_doors' '00012fd5 (/E-STEER Core/SubSystem Specifications/Application Functions - EA4/SF049A Loss of Assist Manager)' '#SF049A_120' 'true' 'REQ:  SF049A_120' '' } %GIDa_246603fb_11d3_47f2_877c_b57e34b65725"  Value=LoaMgrHwTqLoaAvlResp
  Constant5 : Constant  RequirementInfo="{'linktype_rmi_doors' '00012fd5 (/E-STEER Core/SubSystem Specifications/Application Functions - EA4/SF049A Loss of Assist Manager)' '#SF049A_120' 'true' 'REQ:  SF049A_120' '' } %GIDa_663b9133_8906_4576_b8c8_e86bcfd903f9"  Value=LoaMgrHwTqIdptSig0NoTqLoaResp
  CopyRight2 : Subsystem  Description=|  mask(Copyright Information){none=on}
      | Copyright info block.                                               
      |                                                                     
      | Place copyright information at the top of every subsystem in design.
      mask prompts: none "No parameters"
      mask help: Place copyright information at the top of every subsystem in design.
      mask Display:
      | NxtrConf = 'Nexteer Confidential';
      | 
      | sys = bdroot; %handle for the current model ("system")
      | first = get_param(sys,'Created');
      | first = first(end-3:end);  %year is last four digits
      | 
      | last = get_param(sys,'LastModifiedDate');
      | if isempty(last)
      |     last = datestr(now,'yyyy');
      | else
      |     last = last(end-3:end);
      | end
      | 
      | if strcmp(first,last)
      |     fprintf('%s -- Copyright %s Nexteer',NxtrConf,first)
      | else
      |     fprintf('%s -- %s%s- %s Nexteer',NxtrConf,char(169),first,last)
      | end
  Four : Subsystem  RequirementInfo="{'linktype_rmi_doors' '00012fd5 (/E-STEER Core/SubSystem Specifications/Application Functions - EA4/SF049A Loss of Assist Manager)' '#SF049A_120' 'true' 'REQ:  SF049A_120' '' } %GIDa_dce21196_3719_4dfb_8740_60d27e7b3a95"  TreatAsAtomicUnit=on
      settings: RTWSystemCode=Inline
  Merge1 : Merge  RequirementInfo="{'linktype_rmi_doors' '00012fd5 (/E-STEER Core/SubSystem Specifications/Application Functions - EA4/SF049A Loss of Assist Manager)' '#SF049A_120' 'true' 'REQ:  SF049A_120' '' } %GIDa_a7ef1184_fa36_412f_8746_0eb6c43ab061"  Inputs=4
  Switch Case : SwitchCase  RequirementInfo="{'linktype_rmi_doors' '00012fd5 (/E-STEER Core/SubSystem Specifications/Application Functions - EA4/SF049A Loss of Assist Manager)' '#SF049A_120' 'true' 'REQ:  SF049A_120' '' } %GIDa_36786bcd_ccc9_48ca_8ecd_6a29494ce015"  CaseConditions={4,2,1}
  Two : Subsystem  RequirementInfo="{'linktype_rmi_doors' '00012fd5 (/E-STEER Core/SubSystem Specifications/Application Functions - EA4/SF049A Loss of Assist Manager)' '#SF049A_120' 'true' 'REQ:  SF049A_120' '' } %GIDa_30c7ba8f_d98f_43f6_9daa_542d3c7f7f17"  TreatAsAtomicUnit=on
      settings: RTWSystemCode=Inline
  Zero_or_Invalid : Subsystem  RequirementInfo="{'linktype_rmi_doors' '00012fd5 (/E-STEER Core/SubSystem Specifications/Application Functions - EA4/SF049A Loss of Assist Manager)' '#SF049A_120' 'true' 'REQ:  SF049A_120' '' } %GIDa_8d308621_e2ff_4ce2_90d3_e162a34f8e92"  TreatAsAtomicUnit=on
      settings: RTWSystemCode=Inline
  one : Subsystem  RequirementInfo="{'linktype_rmi_doors' '00012fd5 (/E-STEER Core/SubSystem Specifications/Application Functions - EA4/SF049A Loss of Assist Manager)' '#SF049A_120' 'true' 'REQ:  SF049A_120' '' } %GIDa_c5591306_9021_4e88_a104_aaf27cc4691e"  TreatAsAtomicUnit=on
      settings: RTWSystemCode=Inline
  HwTqResp : Outport  RequirementInfo={} %GIDa_f7daceac_6af4_479a_9ffd_0a0d7a37b5c0
  wires:
  Merge1/1 -> HwTqResp/1
  Zero_or_Invalid/1(HwTqResp) -> Merge1/4
  one/1(HwTqResp) -> Merge1/3
  Two/1(HwTqResp) -> Merge1/2
  Four/1(HwTqResp) -> Merge1/1
  [TqLoaAvl] -> Zero_or_Invalid/3(TqLoaAvl)
  Constant5/1 -> Zero_or_Invalid/2(Sig0NoTqLoaResp)
  Constant4/1 -> Zero_or_Invalid/1(TqLoaAvlResp)
  [TqLoaAvl] -> one/3(TqLoaAvl)
  TqLoaAvl/1 -> [TqLoaAvl]
  Constant3/1 -> one/2(Sig1NoTqLoaResp)
  Constant2/1 -> one/1(TqLoaAvlResp)
  Constant1/1 -> Two/1(cal)
  Switch Case/2 -> Two/Action
  Constant/1 -> Four/1(cal)
  Switch Case/1 -> Four/Action
  Switch Case/4 -> Zero_or_Invalid/Action
  HwTqIdptMin/1 -> Switch Case/1
  Switch Case/3 -> one/Action
